simulink model "ModeAdjustCallerForTest"  (R2018b)
settings: Solver=FixedStepDiscrete  StartTime=0.0  StopTime=10.0  FixedStep=0.01  RelTol=1e-3
undefined symbols (not defined in the file): DrvSt_Cal, KeSMSeHeiCstTypeConfig_Val, MdXXIsPosChk_Cal, ModeStEnCtrlCaller_Cal, PassSt_Cal, SecRwLtSt_Cal, SecRwRtSt_Cal, ThdRwLtSt_Cal, ThdRwRtSt_Cal
settings Model: Creator=sn2xws  LastModifiedBy=sn2xws
settings DataIOCC: SaveFormat=StructureWithTime
settings OptimizationCC: DefaultParameterBehavior=Inlined  EnhancedBackFolding=on  PassReuseOutputArgsAs=Individual arguments  ZeroExternalMemoryAtStartup=off  ZeroInternalMemoryAtStartup=off  OptimizeBlockOrder=speed  DifferentSizesBufferReuse=on  OptimizationCustomize=off
settings DebuggingCC: ParameterTunabilityLossMsg=error
settings ModelReferenceCC: ModelReferenceNumInstancesAllowed=Single
settings SFSimCC: MATLABDynamicMemAlloc=off
settings RTWCC: SystemTargetFile=autosar.tlc  GenCodeOnly=on  TemplateMakefile=ert_default_tmf  Description=AUTOSAR  GenerateReport=on  IncludeHyperlinkInReport=on  LaunchReport=on  GenerateTraceInfo=on  GenerateTraceReport=on  GenerateTraceReportSl=on  GenerateTraceReportSf=on  GenerateTraceReportEml=on
settings CodeAppCC: ForceParamTrailComments=on  IgnoreCustomStorageClasses=off  OperatorAnnotations=on  SimulinkDataObjDesc=on  SFDataObjDesc=on  InsertBlockDesc=on
settings STFCustomTargetCC: TargetLangStandard=C99 (ISO)  MultiwordLength=256  ParMdlRefBuildCompliant=on  CompOptLevelCompliant=on  IncludeMdlTerminateFcn=off  CombineOutputUpdateFcns=on  SuppressErrorStatus=on  ERTCustomFileBanners=on  SupportNonFinite=off  SupportComplex=off  SupportContinuousTime=off  SupportNonInlinedSFcns=off  RemoveResetFunc=on  MATLABClassNameForMDSCustomization=Simulink.SoftwareTarget.ERTCustomization  AutosarCompliant=on  UseToolchainInfoCompliant=on  LookupTableObjectStructAxisOrder=2,1,3,4,...  LUTObjectStructOrderEvenSpacing=Size,Table,Breakpoints  SystemTargetFile=autosar.tlc
settings ERTTargetCC: TargetLangStandard=C99 (ISO)  ConcurrentExecutionCompliant=off  IncludeMdlTerminateFcn=off  SuppressErrorStatus=on  SupportNonFinite=off  SupportComplex=off  ModelStepFunctionPrototypeControlCompliant=off  CPPClassGenCompliant=off  AutosarCompliant=on  LookupTableObjectStructAxisOrder=2,1,3,4,...  LUTObjectStructOrderEvenSpacing=Size,Table,Breakpoints  InlinedParameterPlacement=NonHierarchical  ERTCustomFileTemplate=example_file_process.tlc

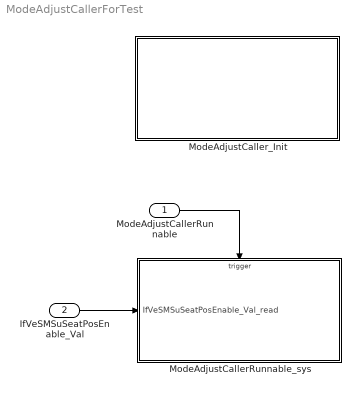
== system ModeAdjustCallerForTest ==
  ModeAdjustCallerRunnable : Inport  SampleTime=0.01  OutputFunctionCall=on
  IfVeSMSuSeatPosEnable_Val : Inport  Port=2  OutDataTypeStr=uint8  PortDimensions=1
  ModeAdjustCallerRunnable_sys : Subsystem
  ModeAdjustCaller_Init : Subsystem
  wires:
  IfVeSMSuSeatPosEnable_Val/1 -> ModeAdjustCallerRunnable_sys/1(IfVeSMSuSeatPosEnable_Val_read)
  ModeAdjustCallerRunnable/1 -> ModeAdjustCallerRunnable_sys/Trigger

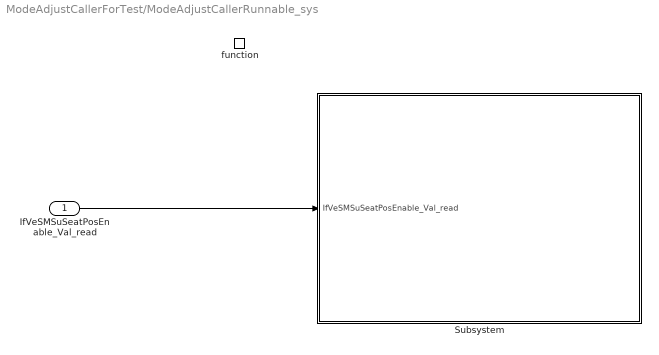
== system ModeAdjustCallerForTest/ModeAdjustCallerRunnable_sys ==
  IfVeSMSuSeatPosEnable_Val_read : Inport
  function : TriggerPort  TriggerType=function-call  VariantControl=(inherit)  SampleTimeType=periodic  SampleTime=-1
  Subsystem : Subsystem
  wires:
  IfVeSMSuSeatPosEnable_Val_read/1 -> Subsystem/1(IfVeSMSuSeatPosEnable_Val_read)

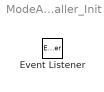
== system ModeAdjustCallerForTest/ModeAdjustCaller_Init ==
  Event Listener : EventListener  EventName=reset

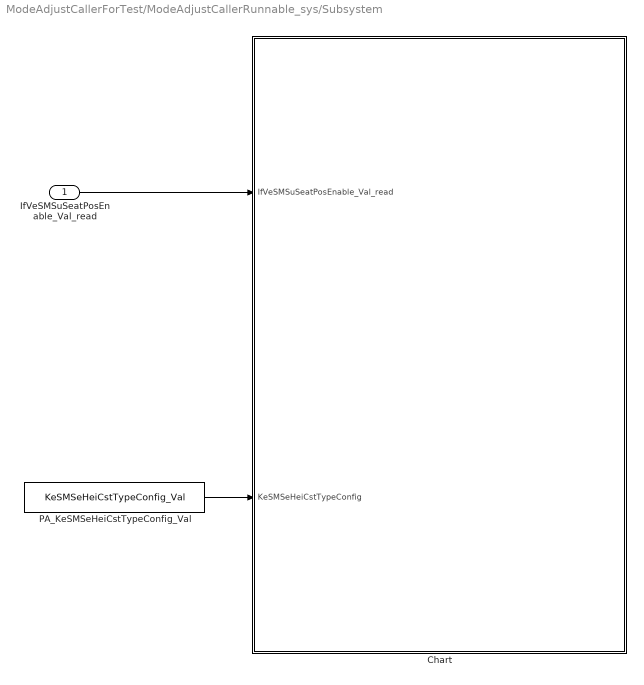
== system ModeAdjustCallerForTest/ModeAdjustCallerRunnable_sys/Subsystem ==
  IfVeSMSuSeatPosEnable_Val_read : Inport
  Chart : Stateflow chart  TreatAsAtomicUnit=on
  PA_KeSMSeHeiCstTypeConfig_Val : Constant  Value=KeSMSeHeiCstTypeConfig_Val
  wires:
  IfVeSMSuSeatPosEnable_Val_read/1 -> Chart/1(IfVeSMSuSeatPosEnable_Val_read)
  PA_KeSMSeHeiCstTypeConfig_Val/1 -> Chart/2(KeSMSeHeiCstTypeConfig)

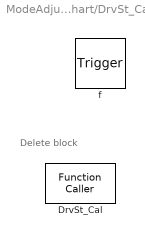
== system ModeAdjustCallerForTest/ModeAdjustCallerRunnable_sys/Subsystem/Chart/DrvSt_Cal ==
  note: Delete block
  f : TriggerPort  TriggerType=function-call  VariantControl=(inherit)
      settings: CopyFcn=Stateflow.SLINSF.SimulinkMan.removeBlockPreDeleteFcn  PreDeleteFcn=Stateflow.SLINSF.SimulinkMan.unsafePredeleteFcn
  DrvSt_Cal : FunctionCaller  FunctionPrototype=DrvSt_Cal()

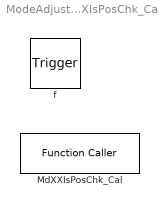
== system ModeAdjustCallerForTest/ModeAdjustCallerRunnable_sys/Subsystem/Chart/MdXXIsPosChk_Cal ==
  f : TriggerPort  TriggerType=function-call  VariantControl=(inherit)
      settings: CopyFcn=Stateflow.SLINSF.SimulinkMan.removeBlockPreDeleteFcn  PreDeleteFcn=Stateflow.SLINSF.SimulinkMan.unsafePredeleteFcn
  MdXXIsPosChk_Cal : FunctionCaller  FunctionPrototype=MdXXIsPosChk_Cal()

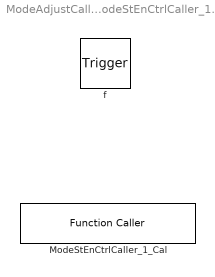
== system ModeAdjustCallerForTest/ModeAdjustCallerRunnable_sys/Subsystem/Chart/ModeStEnCtrlCaller_1_Cal ==
  f : TriggerPort  TriggerType=function-call  VariantControl=(inherit)
      settings: CopyFcn=Stateflow.SLINSF.SimulinkMan.removeBlockPreDeleteFcn  PreDeleteFcn=Stateflow.SLINSF.SimulinkMan.unsafePredeleteFcn
  ModeStEnCtrlCaller_1_Cal : FunctionCaller  FunctionPrototype=ModeStEnCtrlCaller_Cal()

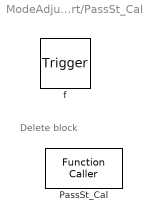
== system ModeAdjustCallerForTest/ModeAdjustCallerRunnable_sys/Subsystem/Chart/PassSt_Cal ==
  note: Delete block
  f : TriggerPort  TriggerType=function-call  VariantControl=(inherit)
      settings: CopyFcn=Stateflow.SLINSF.SimulinkMan.removeBlockPreDeleteFcn  PreDeleteFcn=Stateflow.SLINSF.SimulinkMan.unsafePredeleteFcn
  PassSt_Cal : FunctionCaller  FunctionPrototype=PassSt_Cal()

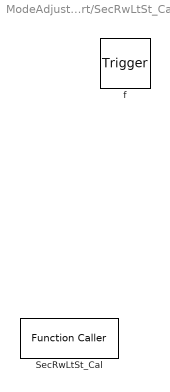
== system ModeAdjustCallerForTest/ModeAdjustCallerRunnable_sys/Subsystem/Chart/SecRwLtSt_Cal ==
  f : TriggerPort  TriggerType=function-call  VariantControl=(inherit)
      settings: CopyFcn=Stateflow.SLINSF.SimulinkMan.removeBlockPreDeleteFcn  PreDeleteFcn=Stateflow.SLINSF.SimulinkMan.unsafePredeleteFcn
  SecRwLtSt_Cal : FunctionCaller  FunctionPrototype=SecRwLtSt_Cal()

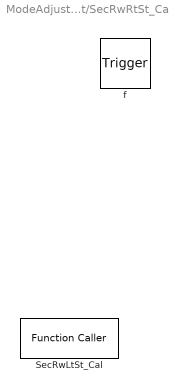
== system ModeAdjustCallerForTest/ModeAdjustCallerRunnable_sys/Subsystem/Chart/SecRwRtSt_Cal ==
  f : TriggerPort  TriggerType=function-call  VariantControl=(inherit)
      settings: CopyFcn=Stateflow.SLINSF.SimulinkMan.removeBlockPreDeleteFcn  PreDeleteFcn=Stateflow.SLINSF.SimulinkMan.unsafePredeleteFcn
  SecRwLtSt_Cal : FunctionCaller  FunctionPrototype=SecRwRtSt_Cal()

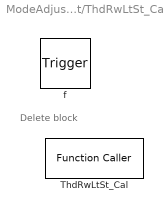
== system ModeAdjustCallerForTest/ModeAdjustCallerRunnable_sys/Subsystem/Chart/ThdRwLtSt_Cal ==
  note: Delete block
  f : TriggerPort  TriggerType=function-call  VariantControl=(inherit)
      settings: CopyFcn=Stateflow.SLINSF.SimulinkMan.removeBlockPreDeleteFcn  PreDeleteFcn=Stateflow.SLINSF.SimulinkMan.unsafePredeleteFcn
  ThdRwLtSt_Cal : FunctionCaller  FunctionPrototype=ThdRwLtSt_Cal()

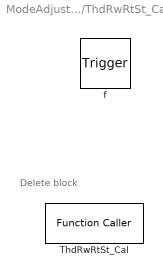
== system ModeAdjustCallerForTest/ModeAdjustCallerRunnable_sys/Subsystem/Chart/ThdRwRtSt_Cal ==
  note: Delete block
  f : TriggerPort  TriggerType=function-call  VariantControl=(inherit)
      settings: CopyFcn=Stateflow.SLINSF.SimulinkMan.removeBlockPreDeleteFcn  PreDeleteFcn=Stateflow.SLINSF.SimulinkMan.unsafePredeleteFcn
  ThdRwRtSt_Cal : FunctionCaller  FunctionPrototype=ThdRwRtSt_Cal()

== stateflow chart ModeAdjustCallerForTest/ModeAdjustCallerRunnable_sys/Subsystem/Chart ==
  state DrvSt_Cal [function]
  state PassSt_Cal [function]
  state SecRwLtSt_Cal [function]
  state SecRwRtSt_Cal [function]
  state ThdRwLtSt_Cal [function]
  state ThdRwRtSt_Cal [function]
  state MdXXIsPosChk_Cal [function]
  state ModeStEnCtrlCaller_1_Cal [function]
  (default) -> (junction 2)
  (junction 2) -> (junction 4) [order 1] : [IfVeSMSuSeatPosEnable_Val_read==4 &&KeSMSeHeiCstTypeConfig==1]
  (junction 2) -> (junction 10) [order 2]
  (junction 4) -> (junction 7) : %{HMIHeightSelc2R_Cal();}
  (junction 7) -> (junction 10)
  (junction 10) -> (junction 13)
  (junction 13) -> (junction 15) [order 1] : [IfVeSMSuSeatPosEnable_Val_read==3 &&KeSMSeHeiCstTypeConfig==1]
  (junction 13) -> (junction 20) [order 2]
  (junction 15) -> (junction 17) : %{HMIHeightSelc2L_Cal();}
  (junction 17) -> (junction 20)
  (junction 20) -> (junction 23)
  (junction 23) -> (junction 25) [order 1] : [IfVeSMSuSeatPosEnable_Val_read==3]
  (junction 23) -> (junction 37) [order 2]
  (junction 25) -> (junction 28) : {
      | DrvSt_Cal();
      | PassSt_Cal();
      | SecRwLtSt_Cal();
      | SecRwRtSt_Cal();
      | ThdRwLtSt_Cal();
      | ThdRwRtSt_Cal();
      | MdXXIsPosChk_Cal();
      | ModeStEnCtrlCaller_1_Cal();
      | }
  (junction 28) -> (junction 37)
  data: IfVeSMSuSeatPosEnable_Val_read input; KeSMSeHeiCstTypeConfig input
